simulink model "ACDCMG_sim8"  (R2019b)
settings: Solver=ode8  StartTime=0.0  StopTime=0.5  FixedStep=40e-6  MaxStep=1e-2  RelTol=1e-3
PreLoadFcn:
  | Set_parameters_R2018
InitFcn:
  | Set_parameters_R2018
values from neighbouring files (symbols this model uses):
  dis11 = 3    [Set_parameters_R2018.m]
  dis12 = 3    [Set_parameters_R2018.m]
  dis2 = 0.2    [Set_parameters_R2018.m]
  dis3 = 0.15    [Set_parameters_R2018.m]
  dis4 = 0.2    [Set_parameters_R2018.m]
  dis5 = 0.25    [Set_parameters_R2018.m]
  dis6 = 0.1    [Set_parameters_R2018.m]
  Fnom = 60    [Set_parameters_R2018.m]
  max_min = 1    [Set_parameters_R2018.m]
  P_Load_3 = S_Load_3* PF_Load_3    (= 7650)    [Set_parameters_R2018.m]
  Pnom_T1 = 1.5e6    (= 1500000)    [Set_parameters_R2018.m]
  Pnom_T2 = 1.5e6    (= 1500000)    [Set_parameters_R2018.m]
  Pnom_T3 = 4e6    (= 4000000)    [Set_parameters_R2018.m]
  Ql_Load_3 = S_Load_3 * sin(acos(PF_Load_3))    [Set_parameters_R2018.m]
  R_Load_9 = (Vnom_prim * 1.35)^2 / P_Load_9    (= 1084.6153125)    [Set_parameters_R2018.m]
  R_Load_DC = Vnom_DC^2/ P_Load_DC    (= 45)    [Set_parameters_R2018.m]
  Rl = 0.17    [Set_parameters_R2018.m]
  Rls = 0.013    [Set_parameters_R2018.m]
  Ts = 40e-6    (= 4e-05)    [Set_parameters_R2018.m]
  Ts_Control = 6*Ts_Power    (= 0.00024)    [Set_parameters_R2018.m]
  Ts_Power = Ts    (= 4e-05)    [Set_parameters_R2018.m]
  Ts_PV = 0.05    [Set_parameters_R2018.m]
  V1_LL_T3 = 69e3    (= 69000)    [Set_parameters_R2018.m]
  Vmin_mppt = 100    [Set_parameters_R2018.m]
  Vnom_DC = 300    [Set_parameters_R2018.m]
  Vnom_Diesel = 2.4e3    (= 2400)    [Set_parameters_R2018.m]
  Vnom_prim = 13.8e3    (= 13800)    [Set_parameters_R2018.m]
  Vnom_sec = 220    [Set_parameters_R2018.m]
  Vnom_ter_AC_DC = 150    [Set_parameters_R2018.m]
  Xl = 0.3    [Set_parameters_R2018.m]
  Xls = 0.93e-3    (= 0.00093)    [Set_parameters_R2018.m]
undefined symbols (not defined in the file or in its folder): D1, Delta, DiscIntNeverNeededParam, fn, Ion, Lithium, VnInv
libraries: powerlib x136, powerlib_meascontrol x67, rtlab x23, artemis x7, simulink x7, powerlib_extras x5, electricdrivelib x1, eeSinusoidalMeasurementV2 x1, op_dpl_lib x1, re_lib x1
(part 4 of 5)

== system ACDCMG_sim8/SM_Grid_Simulation/Boost -buck Bi-directional converter 1/Primary Control ==
  V_ref : Inport
  Constant : Constant
  Display3 : Display  Commented=on
  From1 : From  Commented=on  GotoTag=Vdc_bus  TagVisibility=global
  From4 : From  Commented=on  GotoTag=boost1
  From5 : From  Commented=on  GotoTag=buck1
  PID Orig Boost : Subsystem
  Relational Operator2 : RelationalOperator  Commented=on  Operator=>  OutDataTypeStr=boolean  RndMeth=Nearest
  Saturation : Saturate  UpperLimit=0.9  LowerLimit=0.1
  Sum : Sum  Inputs=|+-
  Sum1 : Sum  Inputs=|-+
  Switch : Switch  Commented=on  Criteria=u2 > Threshold  Threshold=300
  Switch1 : Switch  Commented=on  Criteria=u2 > Threshold  Threshold=300
  Vref1 : Constant  Commented=on  Value=0
  Vref2 : Constant  Commented=on  Value=0
  Duty_Ctrl : Outport  VectorParamsAs1DForOutWhenUnconnected=off
  Comp_Duty_Ctrl : Outport  Port=2  VectorParamsAs1DForOutWhenUnconnected=off
  wires:
  Relational Operator2/1 -> Switch1/2, Switch/2
  V_ref/1 -> Sum/1, Relational Operator2/2
  From1/1 -> Relational Operator2/1
  Vref2/1 -> Switch1/1
  [V_DC_bus_BESS] -> Sum/2
  From5/1 -> Switch/1
  From4/1 -> Switch1/3
  Switch/1 -> Display3/1
  Vref1/1 -> Switch/3
  Sum/1 -> PID Orig Boost/1(error)  "error"
  PID Orig Boost/1(Out1) -> Saturation/1
  Constant/1 -> Sum1/2
  Saturation/1 -> Sum1/1, Duty_Ctrl/1
  Sum1/1 -> Comp_Duty_Ctrl/1

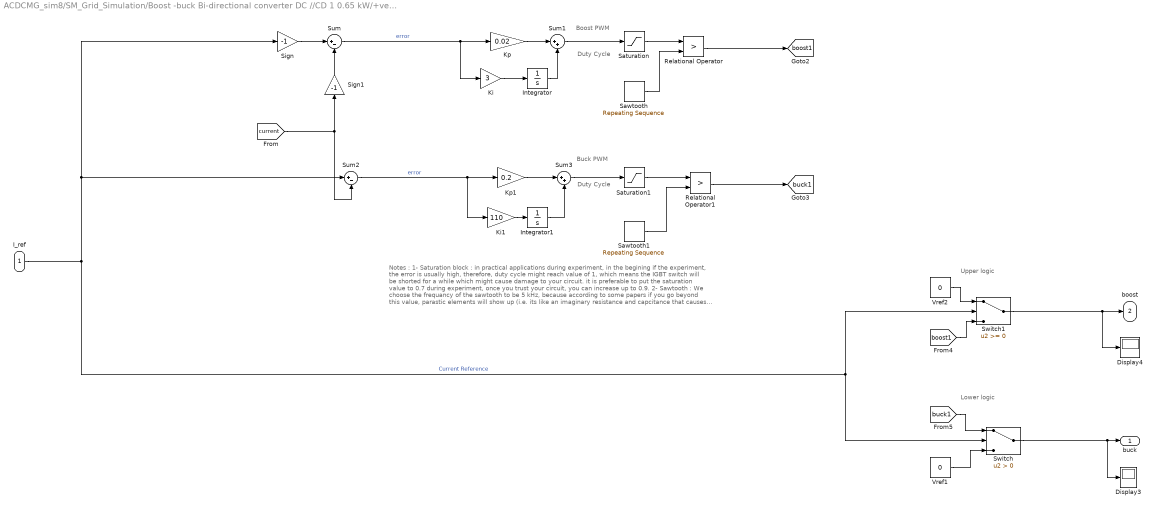
== system ACDCMG_sim8/SM_Grid_Simulation/Boost -buck Bi-directional converter DC //CD 1 0.65 kW/+ve reference For Buck --> -ve reference For Boost <-- ==
  note: Notes :
      | 1- Saturation block : in practical applications during experiment, in the begining if the experiment, the error is usually high, therefore, duty cycle might reach value of 1, which means the IGBT switch will be shorted for a while which might cause damage to your circuit. it is preferable to put the saturation value to 0.7 during experiment, once you trust your circuit, you can increase up to 0.9.
      | 2- Sawtooth : We choose the frequancy of the sawtooth to be 5 kHz, because according to some papers if you go beyond this value, parastic elements will show up (i.e. its like an imaginary resistance and capcitance that causes switching losses and heat). But the more you increase the frequency, the smoother the signal you will get.
      | 3- Step size of your mode l: Make sure that the step size (sample time) in the "model configuration parameters" is smaller than 1/f of the sawtooth. For example, lets say that the sawtooth f = 2 Hz or cycle/sec, meaning the triangle (cycle) repeats every 1/2 sec. Step size or sample time means how many point matlab plot every cycle, lets say it is 1/4 (i.e. plot a point every 0.25 sec), that means that the triangle will be plotted with only two points. That reduce the accuracy, Moreover if the step size is greater than 1/f of the sawtooth, the sawtooth output will be zero.
  note: Buck PWM
  note: Duty Cycle
  note: Upper logic
  note: Lower logic
  note: Boost PWM
  note: Duty Cycle
  I_ref : Inport
  Display3 : Display
  Display4 : Display
  Integrator : Integrator  LimitOutput=on  UpperSaturationLimit=0.9  LowerSaturationLimit=0
  Integrator1 : Integrator  LimitOutput=on  UpperSaturationLimit=0.9  LowerSaturationLimit=0
  Ki : Gain  Gain=3
  Ki1 : Gain  Gain=110
  Kp : Gain  Gain=0.02
  Kp1 : Gain  Gain=0.2
  Relational Operator : RelationalOperator  Operator=>  OutDataTypeStr=boolean  RndMeth=Nearest
  Relational Operator1 : RelationalOperator  Operator=>  OutDataTypeStr=boolean  RndMeth=Nearest
  Saturation : Saturate  UpperLimit=0.9  LowerLimit=0
  Saturation1 : Saturate  UpperLimit=0.8  LowerLimit=0
  Sawtooth : simulink/Sources/Repeating Sequence  rep_seq_t=[0 1/5000]  rep_seq_y=[0 1]
  Sawtooth1 : simulink/Sources/Repeating Sequence  rep_seq_t=[0 1/5000]  rep_seq_y=[0 1]
  Sign : Gain  Gain=-1
  Sign1 : Gain  Gain=-1
  Sum : Sum  Inputs=|+-
  Sum1 : Sum  Inputs=|++
  Sum2 : Sum  Inputs=|+-
  Sum3 : Sum  Inputs=|++
  Switch : Switch  Criteria=u2 > Threshold
  Switch1 : Switch
  Vref1 : Constant  Value=0
  Vref2 : Constant  Value=0
  buck : Outport  VectorParamsAs1DForOutWhenUnconnected=off
  boost : Outport  Port=2  VectorParamsAs1DForOutWhenUnconnected=off
  tag scope: boost1=global, buck1=global
  wires:
  Integrator/1 -> Sum1/2
  Kp/1 -> Sum1/1
  Sum/1 -> Kp/1, Ki/1  "error"
  Relational Operator/1 -> [boost1]
  Sign/1 -> Sum/1
  Sum1/1 -> Saturation/1
  Ki/1 -> Integrator/1
  Sum3/1 -> Saturation1/1
  Integrator1/1 -> Sum3/2
  Sawtooth/1 -> Relational Operator/2
  Sawtooth1/1 -> Relational Operator1/2
  [current] -> Sum2/2, Sign1/1
  Kp1/1 -> Sum3/1
  Relational Operator1/1 -> [buck1]
  Sum2/1 -> Ki1/1, Kp1/1  "error"
  Saturation/1 -> Relational Operator/1
  Saturation1/1 -> Relational Operator1/1
  Ki1/1 -> Integrator1/1
  Vref1/1 -> Switch/3
  Vref2/1 -> Switch1/1
  [boost1] -> Switch1/3
  [buck1] -> Switch/1
  I_ref/1 -> Sum2/1, Sign/1, Switch1/2, Switch/2  "Current Reference"
  Sign1/1 -> Sum/2
  Switch1/1 -> Display4/1, boost/1
  Switch/1 -> Display3/1, buck/1

== system ACDCMG_sim8/SM_Grid_Simulation/Boost -buck Bi-directional converter DC //CD 1 0.65 kW/ref ==
  note: 1 -charge
      | 0-discharge
  Constant2 : Constant  Value=max_min
  Constant3 : Constant  Value=max_min
  Current reference (battery charge) OP_Max : Constant  Value=5
  Current reference (battery discharge) OP_Max1 : Constant  Value=-5
  Min Demand OP_min : Constant  Value=3
  Min Demand OP_min1 : Constant  Value=-3
  Switch : Switch  Criteria=u2 > Threshold
  Switch1 : Switch  Criteria=u2 > Threshold
  Switch3 : Switch  Criteria=u2 > Threshold
  Vref1 : Constant
  ref : Outport  VectorParamsAs1DForOutWhenUnconnected=off
  wires:
  Constant3/1 -> Switch3/2
  Switch3/1 -> Switch/3
  Switch1/1 -> Switch/1
  Vref1/1 -> Switch/2
  Min Demand OP_min/1 -> Switch1/3
  Current reference (battery charge) OP_Max/1 -> Switch1/1
  Min Demand OP_min1/1 -> Switch3/3
  Constant2/1 -> Switch1/2
  Current reference (battery discharge) OP_Max1/1 -> Switch3/1
  Switch/1 -> ref/1

== system ACDCMG_sim8/SM_Grid_Simulation/Boost converter 2 5 kHz - 300V /MPPT Controller using  Incremental Conductance and Integral Regulator  technique  ==
  note: +
  note: control mppt
  V_PV : Inport
  I_PV : Inport  Port=2
  Add : Sum
  Deblock MPPT : Step  Time=Ts_PV  Before=-1  SampleTime=0
  Duty Cycle : Constant  Commented=on  Value=Dinit
  Goto7 : Goto  Commented=on  GotoTag=D  TagVisibility=global
  MPPT : Subsystem
  PWM Generator (DC-DC) : powerlib_meascontrol/Pulse & Signal Generators/PWM Generator (DC-DC)  Commented=on  Fsw=fc  Ts=Ts_Power
  Saturation : Saturate  UpperLimit=0.9  LowerLimit=0.1
  Pulses : Outport  VectorParamsAs1DForOutWhenUnconnected=off
  wires:
  V_PV/1 -> MPPT/1(V_PV)
  I_PV/1 -> MPPT/2(I_PV)
  Deblock MPPT/1 -> MPPT/3(on/off)
  Add/1 -> Saturation/1  "D"
  MPPT/1(D) -> Add/2  "Vdc_ref"
  Saturation/1 -> Pulses/1

== system ACDCMG_sim8/SM_Grid_Simulation/Bus_1/Power Factor Block1 ==
  Vabc : Inport
  Iabc : Inport  Port=2
  Complex to Magnitude-Angle : ComplexToMagnitudeAngle  Commented=on
  Conv pu2 : Gain  Gain=1/Vnom_Diesel  SaturateOnIntegerOverflow=on  OutDataTypeStr=Inherit: Same as input  ParamDataTypeStr=Inherit: Same as input
  Current3 : Goto  Commented=on  GotoTag=P_abc_Bus8  TagVisibility=global
  Current4 : Goto  Commented=on  GotoTag=Q_abc_Bus8  TagVisibility=global
  Gain : Gain  Commented=on  Gain=-1/1000
  Gain1 : Gain  Commented=on  Gain=-1/1000
  Memory : Memory
  Power : powerlib_meascontrol/Measurements/Power  Commented=on  Freq=Freq  Vinit=Vinit  Iinit=Iinit  Ts=Ts
  RMS : powerlib_meascontrol/Measurements/RMS  TrueRMS=on  Freq=60  RMSInit=120  Ts=0
  Real-Imag to Complex : RealImagToComplex  Commented=on
  Terminator : Terminator  Commented=on
  cos(theta) : Trigonometry  Commented=on  Operator=cos
  "Vabc y Vabc " : Outport  VectorParamsAs1DForOutWhenUnconnected=off
  "Iabc y Iabc " : Outport  Port=2  VectorParamsAs1DForOutWhenUnconnected=off
  tag scope: Vabc_LL_pu_Bus1=global
  wires:
  Complex to Magnitude-Angle/2 -> cos(theta)/1
  Real-Imag to Complex/1 -> Complex to Magnitude-Angle/1
  cos(theta)/1 -> ?
  Complex to Magnitude-Angle/1 -> Terminator/1
  Iabc/1 -> "Iabc y Iabc "/1, Power/2
  Vabc/1 -> Memory/1, Power/1
  Power/2 -> Real-Imag to Complex/2, Gain/1
  Power/1 -> Gain1/1, Real-Imag to Complex/1
  Gain/1 -> Current4/1
  Gain1/1 -> Current3/1
  RMS/1 -> Conv pu2/1
  Conv pu2/1 -> [Vabc_LL_pu_Bus1]
  Memory/1 -> RMS/1, "Vabc y Vabc "/1

== system ACDCMG_sim8/SM_Grid_Simulation/Bus_2/Power Factor Block1 ==
  Vabc : Inport
  Iabc : Inport  Port=2
  Complex to Magnitude-Angle : ComplexToMagnitudeAngle  Commented=on
  Conv pu1 : Gain  Gain=1/Vnom_sec  SaturateOnIntegerOverflow=on  OutDataTypeStr=Inherit: Same as input  ParamDataTypeStr=Inherit: Same as input
  Current1 : Goto  Commented=on  GotoTag=P_abc_Bus1  TagVisibility=global
  Current2 : Goto  Commented=on  GotoTag=Q_abc_Bus1  TagVisibility=global
  Gain1 : Gain  Commented=on  Gain=-1/1000
  Memory : Memory
  Mux : Mux  Inputs=1
  Power : powerlib_meascontrol/Measurements/Power  Commented=on  Freq=Freq  Vinit=Vinit  Iinit=Iinit  Ts=Ts
  RMS : powerlib_meascontrol/Measurements/RMS  TrueRMS=on  Freq=60  RMSInit=120  Ts=0
  Real-Imag to Complex : RealImagToComplex  Commented=on
  Terminator : Terminator  Commented=on
  cos(theta) : Trigonometry  Commented=on  Operator=cos
  to Kw : Gain  Commented=on  Gain=-1/1000
  "Vabc y Vabc " : Outport  VectorParamsAs1DForOutWhenUnconnected=off
  "Iabc y Iabc " : Outport  Port=2  VectorParamsAs1DForOutWhenUnconnected=off
  tag scope: Vabc_LL_pu_Bus2=global
  wires:
  Power/1 -> Gain1/1, Real-Imag to Complex/1
  Power/2 -> Real-Imag to Complex/2, to Kw/1
  Complex to Magnitude-Angle/2 -> cos(theta)/1
  Real-Imag to Complex/1 -> Complex to Magnitude-Angle/1
  Complex to Magnitude-Angle/1 -> Terminator/1
  Iabc/1 -> "Iabc y Iabc "/1, Power/2
  Mux/1 -> "Vabc y Vabc "/1
  Vabc/1 -> Power/1, Memory/1
  to Kw/1 -> Current2/1
  Gain1/1 -> Current1/1
  RMS/1 -> Conv pu1/1
  Conv pu1/1 -> [Vabc_LL_pu_Bus2]
  Memory/1 -> Mux/1, RMS/1

== system ACDCMG_sim8/SM_Grid_Simulation/Bus_3/Power Factor Block1 ==
  Vabc : Inport
  Iabc : Inport  Port=2
  Complex to Magnitude-Angle : ComplexToMagnitudeAngle  Commented=on
  Conv pu1 : Gain  Gain=1/Vnom_sec  SaturateOnIntegerOverflow=on  OutDataTypeStr=Inherit: Same as input  ParamDataTypeStr=Inherit: Same as input
  Current3 : Goto  Commented=on  GotoTag=P_abc_Bus4  TagVisibility=global
  Current4 : Goto  Commented=on  GotoTag=Q_abc_Bus4  TagVisibility=global
  Memory : Memory
  Mux : Mux  Inputs=1
  Power : powerlib_meascontrol/Measurements/Power  Commented=on  Freq=Freq  Vinit=Vinit  Iinit=Iinit  Ts=Ts
  RMS : powerlib_meascontrol/Measurements/RMS  TrueRMS=on  Freq=60  RMSInit=120  Ts=0
  Real-Imag to Complex : RealImagToComplex  Commented=on
  Terminator : Terminator  Commented=on
  cos(theta) : Trigonometry  Commented=on  Operator=cos
  to Kw : Gain  Commented=on  Gain=1/1000
  to Kw1 : Gain  Commented=on  Gain=1/1000
  Vabc y Vabc : Outport  VectorParamsAs1DForOutWhenUnconnected=off
  "Iabc y Iabc " : Outport  Port=2  VectorParamsAs1DForOutWhenUnconnected=off
  tag scope: Vabc_LL_pu_Bus3=global
  wires:
  Complex to Magnitude-Angle/2 -> cos(theta)/1
  Real-Imag to Complex/1 -> Complex to Magnitude-Angle/1
  cos(theta)/1 -> ?
  Complex to Magnitude-Angle/1 -> Terminator/1
  Iabc/1 -> "Iabc y Iabc "/1, Power/2
  Mux/1 -> Vabc y Vabc/1
  Vabc/1 -> Power/1, Memory/1
  Power/2 -> Real-Imag to Complex/2, to Kw/1
  Power/1 -> to Kw1/1, Real-Imag to Complex/1
  to Kw/1 -> Current4/1
  to Kw1/1 -> Current3/1
  RMS/1 -> Conv pu1/1
  Conv pu1/1 -> [Vabc_LL_pu_Bus3]
  Memory/1 -> Mux/1, RMS/1

== system ACDCMG_sim8/SM_Grid_Simulation/Bus_4/Power Factor Block1 ==
  Vabc : Inport
  Iabc : Inport  Port=2
  Complex to Magnitude-Angle : ComplexToMagnitudeAngle  Commented=on
  Conv pu1 : Gain  Gain=1/Vnom_sec  SaturateOnIntegerOverflow=on  OutDataTypeStr=Inherit: Same as input  ParamDataTypeStr=Inherit: Same as input
  Current3 : Goto  Commented=on  GotoTag=P_abc_Bus4  TagVisibility=global
  Current4 : Goto  Commented=on  GotoTag=Q_abc_Bus4  TagVisibility=global
  Memory : Memory
  Mux : Mux  Inputs=1
  Power : powerlib_meascontrol/Measurements/Power  Commented=on  Freq=Freq  Vinit=Vinit  Iinit=Iinit  Ts=Ts
  RMS : powerlib_meascontrol/Measurements/RMS  TrueRMS=on  Freq=60  RMSInit=120  Ts=0
  Real-Imag to Complex : RealImagToComplex  Commented=on
  Terminator : Terminator  Commented=on
  cos(theta) : Trigonometry  Commented=on  Operator=cos
  to Kw : Gain  Commented=on  Gain=1/1000
  to Kw1 : Gain  Commented=on  Gain=1/1000
  Vabc y Vabc : Outport  VectorParamsAs1DForOutWhenUnconnected=off
  "Iabc y Iabc " : Outport  Port=2  VectorParamsAs1DForOutWhenUnconnected=off
  tag scope: Vabc_LL_pu_Bus4=global
  wires:
  Complex to Magnitude-Angle/2 -> cos(theta)/1
  Real-Imag to Complex/1 -> Complex to Magnitude-Angle/1
  cos(theta)/1 -> ?
  Complex to Magnitude-Angle/1 -> Terminator/1
  Iabc/1 -> "Iabc y Iabc "/1, Power/2
  Mux/1 -> Vabc y Vabc/1
  Vabc/1 -> Power/1, Memory/1
  Power/2 -> Real-Imag to Complex/2, to Kw/1
  Power/1 -> to Kw1/1, Real-Imag to Complex/1
  to Kw/1 -> Current4/1
  to Kw1/1 -> Current3/1
  RMS/1 -> Conv pu1/1
  Conv pu1/1 -> [Vabc_LL_pu_Bus4]
  Memory/1 -> Mux/1, RMS/1

== system ACDCMG_sim8/SM_Grid_Simulation/Bus_5/Power Factor Block1 ==
  Vabc : Inport
  Iabc : Inport  Port=2
  Complex to Magnitude-Angle : ComplexToMagnitudeAngle  Commented=on
  Conv pu1 : Gain  Gain=1/Vnom_sec  SaturateOnIntegerOverflow=on  OutDataTypeStr=Inherit: Same as input  ParamDataTypeStr=Inherit: Same as input
  Current3 : Goto  Commented=on  GotoTag=P_abc_Bus5  TagVisibility=global
  Current4 : Goto  Commented=on  GotoTag=Q_abc_Bus5  TagVisibility=global
  Memory : Memory
  Mux : Mux  Inputs=2
  Power : powerlib_meascontrol/Measurements/Power  Commented=on  Freq=Freq  Vinit=Vinit  Iinit=Iinit  Ts=Ts
  RMS : powerlib_meascontrol/Measurements/RMS  TrueRMS=on  Freq=60  RMSInit=120  Ts=0
  Real-Imag to Complex : RealImagToComplex  Commented=on
  Terminator : Terminator  Commented=on
  cos(theta) : Trigonometry  Commented=on  Operator=cos
  to Kw : Gain  Commented=on  Gain=1/1000
  to Kw1 : Gain  Commented=on  Gain=1/1000
  Vabc y Vabc : Outport  VectorParamsAs1DForOutWhenUnconnected=off
  "Iabc y Iabc " : Outport  Port=2  VectorParamsAs1DForOutWhenUnconnected=off
  tag scope: Vabc_LL_pu_Bus5=global
  wires:
  Complex to Magnitude-Angle/2 -> cos(theta)/1
  Real-Imag to Complex/1 -> Complex to Magnitude-Angle/1
  cos(theta)/1 -> ?
  Complex to Magnitude-Angle/1 -> Terminator/1
  Iabc/1 -> "Iabc y Iabc "/1, Power/2
  Mux/1 -> Vabc y Vabc/1
  Vabc/1 -> Power/1, Memory/1
  Power/2 -> Real-Imag to Complex/2, to Kw/1
  Power/1 -> to Kw1/1, Real-Imag to Complex/1
  to Kw/1 -> Current4/1
  to Kw1/1 -> Current3/1
  RMS/1 -> Conv pu1/1
  Conv pu1/1 -> [Vabc_LL_pu_Bus5]
  Memory/1 -> RMS/1, Mux/2

== system ACDCMG_sim8/SM_Grid_Simulation/Bus_6/Power Factor Block1 ==
  Vabc : Inport
  Iabc : Inport  Port=2
  Complex to Magnitude-Angle : ComplexToMagnitudeAngle  Commented=on
  Conv pu1 : Gain  Gain=1/Vnom_sec  SaturateOnIntegerOverflow=on  OutDataTypeStr=Inherit: Same as input  ParamDataTypeStr=Inherit: Same as input
  Current3 : Goto  Commented=on  GotoTag=P_abc_Bus2  TagVisibility=global
  Current4 : Goto  Commented=on  GotoTag=Q_abc_Bus2  TagVisibility=global
  Memory : Memory
  Mux : Mux  Inputs=1
  Power : powerlib_meascontrol/Measurements/Power  Commented=on  Freq=Freq  Vinit=Vinit  Iinit=Iinit  Ts=Ts
  RMS : powerlib_meascontrol/Measurements/RMS  TrueRMS=on  Freq=60  RMSInit=120  Ts=0
  Real-Imag to Complex : RealImagToComplex  Commented=on
  Terminator : Terminator  Commented=on
  cos(theta) : Trigonometry  Commented=on  Operator=cos
  to Kw : Gain  Commented=on  Gain=-1/1000
  to Kw1 : Gain  Commented=on  Gain=-1/1000
  "Vabc y Vabc " : Outport  VectorParamsAs1DForOutWhenUnconnected=off
  Iabc y Iabc : Outport  Port=2  VectorParamsAs1DForOutWhenUnconnected=off
  tag scope: Vabc_LL_pu_Bus6=global
  wires:
  Complex to Magnitude-Angle/2 -> cos(theta)/1
  Real-Imag to Complex/1 -> Complex to Magnitude-Angle/1
  cos(theta)/1 -> ?
  Complex to Magnitude-Angle/1 -> Terminator/1
  Iabc/1 -> Iabc y Iabc/1, Power/2
  Mux/1 -> "Vabc y Vabc "/1
  Vabc/1 -> Power/1, Memory/1
  Power/1 -> to Kw1/1, Real-Imag to Complex/1
  Power/2 -> to Kw/1, Real-Imag to Complex/2
  to Kw/1 -> Current4/1
  to Kw1/1 -> Current3/1
  RMS/1 -> Conv pu1/1
  Conv pu1/1 -> [Vabc_LL_pu_Bus6]
  Memory/1 -> Mux/1, RMS/1

== system ACDCMG_sim8/SM_Grid_Simulation/Bus_7/Power Factor Block1 ==
  Vabc : Inport
  Iabc : Inport  Port=2
  Complex to Magnitude-Angle : ComplexToMagnitudeAngle  Commented=on
  Conv pu1 : Gain  Gain=1/Vnom_sec  SaturateOnIntegerOverflow=on  OutDataTypeStr=Inherit: Same as input  ParamDataTypeStr=Inherit: Same as input
  Memory : Memory
  Power : powerlib_meascontrol/Measurements/Power  Commented=on  Freq=Freq  Vinit=Vinit  Iinit=Iinit  Ts=Ts
  RMS : powerlib_meascontrol/Measurements/RMS  TrueRMS=on  Freq=60  RMSInit=120  Ts=0
  Real-Imag to Complex : RealImagToComplex  Commented=on
  Terminator : Terminator  Commented=on
  cos(theta) : Trigonometry  Commented=on  Operator=cos
  Vabc y Vabc : Outport  VectorParamsAs1DForOutWhenUnconnected=off
  "Iabc y Iabc " : Outport  Port=2  VectorParamsAs1DForOutWhenUnconnected=off
  tag scope: Vabc_LL_pu_Bus7=global
  wires:
  Power/1 -> Real-Imag to Complex/1
  Power/2 -> Real-Imag to Complex/2
  Complex to Magnitude-Angle/2 -> cos(theta)/1
  Real-Imag to Complex/1 -> Complex to Magnitude-Angle/1
  cos(theta)/1 -> ?
  Complex to Magnitude-Angle/1 -> Terminator/1
  Iabc/1 -> "Iabc y Iabc "/1, Power/2
  Vabc/1 -> Memory/1, Power/1
  RMS/1 -> Conv pu1/1
  Conv pu1/1 -> [Vabc_LL_pu_Bus7]
  Memory/1 -> RMS/1, Vabc y Vabc/1

== system ACDCMG_sim8/SM_Grid_Simulation/Bus_8/Power Factor Block1 ==
  Vabc : Inport
  Iabc : Inport  Port=2
  Complex to Magnitude-Angle : ComplexToMagnitudeAngle  Commented=on
  Conv pu1 : Gain  Gain=1/Vnom_ter_AC_DC  SaturateOnIntegerOverflow=on  OutDataTypeStr=Inherit: Same as input  ParamDataTypeStr=Inherit: Same as input
  Memory1 : Memory
  Power : powerlib_meascontrol/Measurements/Power  Commented=on  Freq=Freq  Vinit=Vinit  Iinit=Iinit  Ts=Ts
  RMS : powerlib_meascontrol/Measurements/RMS  TrueRMS=on  Freq=60  RMSInit=120  Ts=0
  Real-Imag to Complex : RealImagToComplex  Commented=on
  Terminator : Terminator  Commented=on
  cos(theta) : Trigonometry  Commented=on  Operator=cos
  "Vabc y Vabc " : Outport  VectorParamsAs1DForOutWhenUnconnected=off
  "Iabc y Iabc " : Outport  Port=2  VectorParamsAs1DForOutWhenUnconnected=off
  tag scope: Vabc_LL_pu_Bus8=global
  wires:
  Power/1 -> Real-Imag to Complex/1
  Power/2 -> Real-Imag to Complex/2
  Complex to Magnitude-Angle/2 -> cos(theta)/1
  Real-Imag to Complex/1 -> Complex to Magnitude-Angle/1
  cos(theta)/1 -> ?
  Complex to Magnitude-Angle/1 -> Terminator/1
  Iabc/1 -> "Iabc y Iabc "/1, Power/2
  Vabc/1 -> Memory1/1, Power/1
  RMS/1 -> Conv pu1/1
  Conv pu1/1 -> [Vabc_LL_pu_Bus8]
  Memory1/1 -> "Vabc y Vabc "/1, RMS/1

== system ACDCMG_sim8/SM_Grid_Simulation/Bus_AC//DC3/Battery system ==
  note: DC Bus (port)
  note: Battery (port)
  "0 = Enable (Do it after transient, so that it does not calculate ripples during transient) 1 = Reset after every change in current reference" : Constant  Commented=on  Value=0
  Current Inst : Scope
  Current going to/ from the battery : Scope
  Mean : powerlib_meascontrol/Measurements/Mean  Freq=10  Vinit=0  Ts=Ts_Power
  Power : Product
  Power Bess1 : Scope
  Power Bus : Scope
  Power1 : Product
  Ripple Calculations : Subsystem  Commented=on
  Ripple in Boost : Display  Commented=on
  Ripple in Buck : Display  Commented=on
  Vbat : Scope
  Vdc : Scope
  to Kw : Gain  Gain=1/1000
  to Kw1 : Gain  Gain=1/1000
  tag scope: DC_Bus_Power=global, Ibat=global, Power_Bess1=global, Vbat=global
  wires:
  to Kw/1 -> [DC_Bus_Power], Power Bus/1
  Mean/1 -> Power/2
  Power/1 -> to Kw/1
  Ripple Calculations/1(Ripple in Buck) -> Ripple in Buck/1
  "0 = Enable (Do it after transient, so that it does not calculate ripples during transient) 1 = Reset after every change in current reference"/1 -> Ripple Calculations/2(Reset)
  Ripple Calculations/2(Ripple in Boost) -> Ripple in Boost/1
  [I_DC_bus_BESS] -> Current Inst/1, Mean/1, Ripple Calculations/1(Signal)
  [Idc_battery] -> Power1/2, [Ibat], Current going to/ from the battery/1
  [V_DC_bus_BESS] -> Vdc/1, Power/1
  [Vdc_battery] -> Power1/1, [Vbat], Vbat/1
  to Kw1/1 -> [Power_Bess1], Power Bess1/1
  Power1/1 -> to Kw1/1

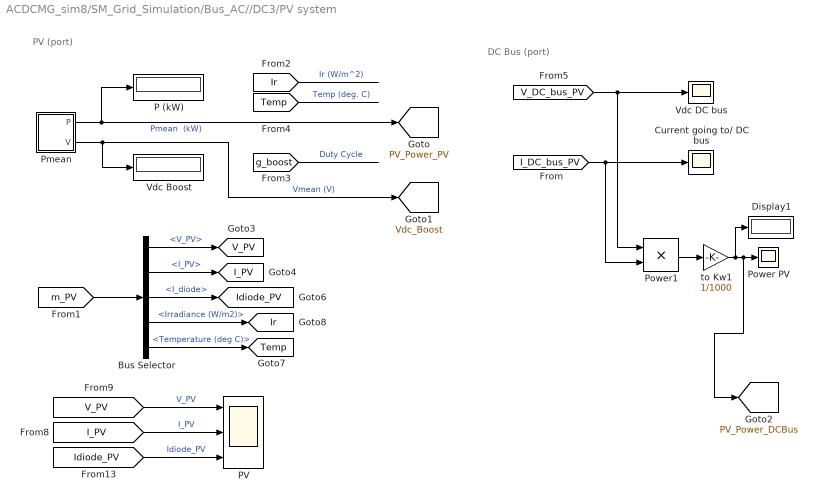
== system ACDCMG_sim8/SM_Grid_Simulation/Bus_AC//DC3/PV system ==
  note: PV (port)
  note: DC Bus (port)
  Bus Selector : BusSelector  OutputSignals=V_PV,I_PV,I_diode,Irradiance (W/m2),Temperature (deg C)
  Current going to/ DC bus : Scope
  Display1 : Display
  "P (kW) " : Display
      settings: Format=bank  Decimation=2000
  PV : Scope  NumInputPorts=3
  Pmean : Subsystem
  Power PV : Scope
  Power1 : Product
  Vdc Boost : Display
      settings: Format=bank  Decimation=2000
  Vdc DC bus : Scope
  to Kw1 : Gain  Gain=1/1000
  tag scope: I_PV=global, Idiode_PV=global, Ir=global, PV_Power_DCBus=global, PV_Power_PV=global, Temp=global, V_PV=global, Vdc_Boost=global
  wires:
  [V_PV] -> PV/1  "V_PV"
  [I_PV] -> PV/2  "I_PV"
  [Idiode_PV] -> PV/3  "Idiode_PV"
  [m_PV] -> Bus Selector/1
  Bus Selector/1 -> [V_PV]  "<V_PV>"
  Bus Selector/2 -> [I_PV]  "<I_PV>"
  Bus Selector/4 -> [Ir]  "<Irradiance (W/m2)>"
  Bus Selector/3 -> [Idiode_PV]  "<I_diode>"
  Bus Selector/5 -> [Temp]  "<Temperature (deg C)>"
  [Temp] -> ?  "Temp (deg. C)"
  [g_boost] -> ?  "Duty Cycle"
  Pmean/2(V) -> [Vdc_Boost], Vdc Boost/1  "Vmean (V)"
  [Ir] -> ?  "Ir (W/m^2)"
  Pmean/1(P) -> [PV_Power_PV], "P (kW) "/1  "Pmean  (kW)"
  [V_DC_bus_PV] -> Vdc DC bus/1, Power1/1
  [I_DC_bus_PV] -> Power1/2, Current going to/ DC bus/1
  to Kw1/1 -> Display1/1, [PV_Power_DCBus], Power PV/1
  Power1/1 -> to Kw1/1

== system ACDCMG_sim8/SM_Grid_Simulation/DATA  ADQUISITION/Power_Losses_abc ==
  From10 : From  Commented=on  GotoTag=Power_Losse_abc_L10  TagVisibility=global
  From11 : From  Commented=on  GotoTag=Power_Losse_abc_L10
  From12 : From  Commented=on  GotoTag=Power_Losse_abc_L12
  From13 : From  Commented=on  GotoTag=Power_Losse_abc_L14
  From6 : From  Commented=on  GotoTag=Power_Losse_abc_L3  TagVisibility=global
  From8 : From  Commented=on  GotoTag=Power_Losse_abc_L8  TagVisibility=global
  From9 : From  Commented=on  GotoTag=Power_Losse_abc_L9  TagVisibility=global
  Mux : Mux  Inputs=7
  f2 : ToWorkspace  VariableName=Power_Losse_abc  SaveFormat=Timeseries  SampleTime=-1
  wires:
  [Power_Losse_abc_L1] -> Mux/1
  Mux/1 -> f2/1
  [Power_Losse_abc_L2] -> Mux/2
  [Power_Losse_abc_L5] -> Mux/5
  [Power_Losse_abc_L6] -> Mux/6
  [Power_Losse_abc_L7] -> Mux/7
  [Power_Losse_abc_L3] -> Mux/3
  [Power_Losse_abc_L4] -> Mux/4

== system ACDCMG_sim8/SM_Grid_Simulation/DATA  ADQUISITION/VoltageLL_pu_abc ==
  From25 : From  Commented=on  GotoTag=Vabc_LL_pu_Bus9  TagVisibility=global
  From28 : From  Commented=on  GotoTag=Vabc_LL_pu_Bus10
  From31 : From  Commented=on  GotoTag=Vabc_LL_pu_Bus10
  From34 : From  Commented=on  GotoTag=Vabc_LL_pu_Bus12
  From40 : From  Commented=on  GotoTag=Vabc_LL_pu_Bus14
  Mux : Mux  Inputs=9
  f2 : ToWorkspace  VariableName=VoltageLL_pu_abc  SaveFormat=Timeseries  SampleTime=-1
  wires:
  [Vabc_LL_pu_Bus4] -> Mux/4
  [Vabc_LL_pu_Bus5] -> Mux/5
  Mux/1 -> f2/1
  [Vabc_LL_pu_Bus8] -> Mux/8
  [Vabc_LL_pu_Bus1] -> Mux/1
  [Vabc_LL_pu_Bus2] -> Mux/2
  [Vabc_LL_pu_Bus6] -> Mux/6
  [Vabc_LL_pu_Bus7] -> Mux/7
  [V_pu_BusDC] -> Mux/9
  [Vabc_LL_pu_Bus3] -> Mux/3

== system ACDCMG_sim8/SM_Grid_Simulation/Grid Bi-directional Converter 1.1 300 (DC) // 150 V (AC) P_nom 3kW2/Control of Inverter ==
  note: VL-L rms_1
  note: Primary control
  note: Control of Inverter
  Means : Inport
  Bus Selector : BusSelector  OutputSignals=signal1,signal2,signal3,signal4
  Discrete PWM Generator1 : Subsystem  AncestorBlock=|  DialogController=POWERSYS.PowerSysDialog  mask(Discrete PWM Generator){GeneratorMode=3-arm  bridge (6 pulses), Fc=4000, Ts=Ts_Power, Internal=off, mIndex=0.99, Freq=60, Phase=0}
      | powerlib_extras/Discrete 
      | Control Blocks/Discrete
      | PWM Generator
      mask prompts: GeneratorMode "Generator Mode"; Fc "Carrier frequency (Hz):"; Ts "Sample time:"; Internal "Internal generation of modulating signal(s)"; mIndex "Modulation index  (0<m<1) :"; Freq "Frequency of output voltage (Hz)"; Phase "Phase of output voltage (degrees)"
      mask help:
      | This discrete block generates pulses for carrier-based PWM (Pulse Width Modulation), self-commutated IGBTs,GTOs or FETs bridges.
      |
      | Depending on the number of bridge arms selected in the "Generator Mode" parameter, the block can be used either for single-phase or three-phase PWM control.
      mask init:
      | powericon('psbcallbacks',gcb,'Discrete PWM Generator');
      | if Freq==0
      |     Phase=90;
      | end
      | switch GeneratorMode
      | case 1,
      |     Internal_Phase=0;
      |    Signal_PortWidth=1;
      |    Select1_Elements=[1 2];
      |    Select1_PortWidth=2;
      |    Select3_Elements=[1 2];
      |    Select3_PortWidth=4;
      | case 2,
      |     Internal_Phase=0;
      |     Signal_PortWidth=1;
      |     Select1_Elements=[1 2];
      |     Select1_PortWidth=2;
      |     Select3_Elements=[1 2 3 4];
      |     Select3_PortWidth=4;
      | case 3,
      |     Internal_Phase=[0 -2*pi/3 2*pi/3];
      |     Signal_PortWidth=3;
      |     Select1_Elements=[1 4 2 5 3 6];
      |     Select1_PortWidth=6;
      |    Select3_Elements=[1 2 3 4 5 6];
      |    Select3_PortWidth=12;
      | case 4,
      |     Internal_Phase=[0 -2*pi/3 2*pi/3];
      |     Signal_PortWidth=3;
      |     Select1_Elements=[1 4 2 5 3 6];
      |     Select1_PortWidth=6;
      |    Select3_Elements=[1 2 3 4 5 6 7 8 9 10 11 12];
      |    Select3_PortWidth=12;
      | end
      | power_initmask();
      mask Help:
      | The output pulses are a vector (with values=0 or 1). Depending on the selected "Generator Mode", the output vector contains:
      | For a 1-arm  bridge: Two pulses. Pulse 1 is for the upper switch and pulse 2 is for the lower switch.
      | For a 2-arm  bridge: Four pulses. Pulses 1 and 3 are respectively for the upper switches of the first and second arm. Pulses 2 and 4 are for the lower switches.
      | For a 3-arm  bridge: Six pulses. Pulses 1,3 and 5 are respectively for the upper switches of the first,second and third arm. Pulses 2,4 and 6 are for the lower switches.
      | For double 3-arm bridges: Twelve pulses.The first six pulses (pulses 1 to 6) must be sent to the first 3-arm bridge and the last six (pulses 7 to 12) to the second 3-arm bridge.
      | 
      | By selecting "Internal generation" you can can control the modulation index m, frequency and phase of the output voltage  from the internal parameters (m, Freq and Phase). Otherwise, external signals are used for pulse generation. The width of the input vector must be 1 for single phase bridges ( 1-arm or 2-arm)  and 3 for 3-phase bridges  (single or double bridge).
      mask TypeOptions GeneratorMode: 1-arm  bridge (2 pulses) | 2-arm  bridge (4 pulses) | 3-arm  bridge (6 pulses) | Double 3-arm  bridges (12 pulses)
      mask Callback Internal: powericon('psbcallbacks',gcb,'Discrete PWM Generator',[]);
  MI Controller : Subsystem
  Unit Delay4 : UnitDelay  SampleTime=Ts_Power  HasFrameUpgradeWarning=on
  VL-L_1 : Scope  NumInputPorts=2
  Vph_abc : Scope
  Vph_rms_1 : Scope
  u / m : Scope
  Pulses : Outport  VectorParamsAs1DForOutWhenUnconnected=off
  wires:
  MI Controller/2(u / m) -> u / m/1
  Unit Delay4/1 -> Pulses/1
  Discrete PWM Generator1/1(Pulses) -> Unit Delay4/1
  Bus Selector/1 -> Vph_abc/1, MI Controller/1(Vabc)  "<signal1>"
  Bus Selector/2 -> VL-L_1/1  "<signal2>"
  Bus Selector/3 -> VL-L_1/2  "<signal3>"
  Bus Selector/4 -> Vph_rms_1/1  "<signal4>"
  Means/1 -> Bus Selector/1
  MI Controller/1(Vabc_inv) -> Discrete PWM Generator1/1(Uref)

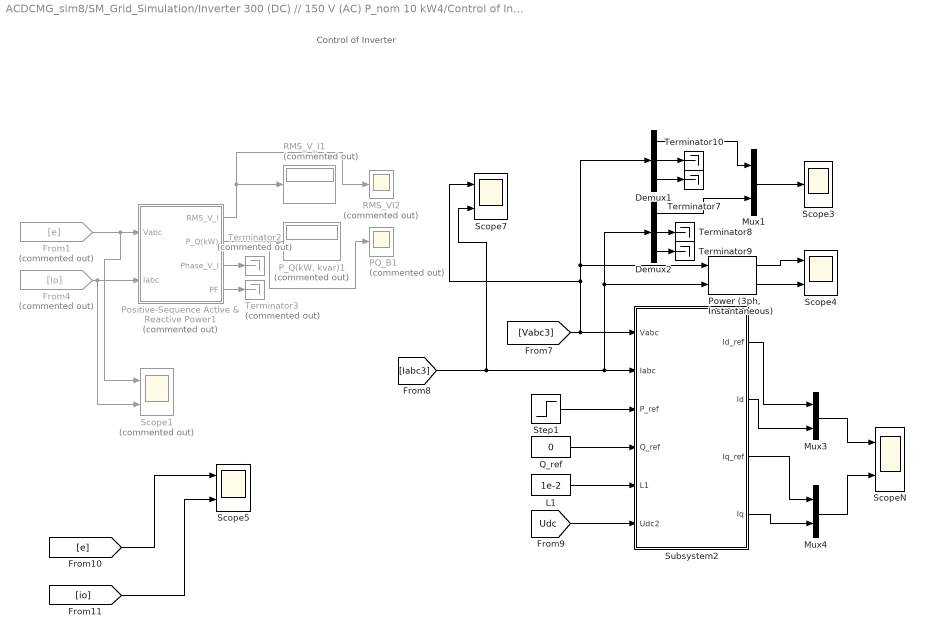
== system ACDCMG_sim8/SM_Grid_Simulation/Inverter 300 (DC) // 150 V (AC) P_nom 10 kW4/Control of Inverter ==
  note: Control of Inverter
  Demux1 : Demux  Outputs=3
  Demux2 : Demux  Outputs=3
  From1 : From  Commented=on  GotoTag=e
      settings: CloseFcn=tagdialog Close
  From4 : From  Commented=on  GotoTag=io
      settings: CloseFcn=tagdialog Close
  L1 : Constant  Value=1e-2
  Mux1 : Mux  Inputs=2
  Mux3 : Mux  Inputs=2
  Mux4 : Mux  Inputs=2
  PQ_B1 : Scope  Commented=on
  "P_Q(kW, kvar)1" : Display  Commented=on
      settings: Format=bank  Decimation=2000
  Positive-Sequence Active & Reactive Power1 : Subsystem  Commented=on  AncestorBlock=|  DialogController=POWERSYS.PowerSysDialog  mask(Discrete 3-phase Positive-Sequence Active & Reactive Power){Freq=60, Par_Vinit=[0 0], Par_Iinit=[0 0], Ts=5e-6}
      | powerlib_extras/Discrete
      | Measurements/Discrete 3-phase 
      | Positive-Sequence 
      | Active & Reactive Power
      mask prompts: Freq "Fundamental frequency (Hz):"; Par_Vinit "Voltage initial input: [ Mag  Phase(degrees) ]"; Par_Iinit "Current initial input: [ Mag  Phase(degrees) ]"; Ts "Sample time:"
      mask help:
      | Measure the three-phase active power P and reactive power Q associated with a periodic set of three-phase voltages and currents which may contain harmonics. P and Q are calculated by evaluating the fundamental values (positive-sequence) of the input voltages and currents with a running window over one cycle of the fundamental frequency.
      |
      | Current flowing into an RL circuit will produce  positive active and reactive powers.
      |
      | Vabc input: Three-phase instantaneous voltage (V)
      | Iabc input: Three-phase instantaneous current (A)
      |
      | Output 1: Vector [Mag_V(V) Mag_I(A)] of the fundamental values of the voltage & current (peak values of the positive-sequence)
      | Output 2: 3-phase PQ measurement vector [P(W) Q (var)] evaluated at the fundamental frequency.
      |
      | For the first cycle of simulation, the outputs are held constant using the values specified by the parameters "Initial input".
      mask init:
      | power_initmask();
      mask Help: This block is part of a subset of blocks in the Extras library that does not have documentation associated with it, other than the block mask description.
      mask Display: disp('')
  "Power (3ph, Instantaneous)" : powerlib_meascontrol/Measurements/Power (3ph, Instantaneous)
  Q_ref : Constant  Value=0
  RMS_VI2 : Scope  Commented=on
  RMS_V_I1 : Display  Commented=on
      settings: Format=bank  Decimation=2000
  Scope1 : Scope  Commented=on  NumInputPorts=2
  Scope3 : Scope
  Scope4 : Scope  NumInputPorts=2
  Scope5 : Scope  NumInputPorts=2
  Scope7 : Scope  NumInputPorts=2
  ScopeN : Scope  NumInputPorts=2
  Step1 : Step  Time=0.07  After=15e3  SampleTime=0
  Subsystem2 : Subsystem  mask{Kp=100, Ki=101, Kd=0}
      mask prompts: Kp "Proportional gain (Kp):"; Ki "Integral gain (Ki):"; Kd "Derivative gain (Kd):"
  Terminator{7..10} (4 alike) : Terminator
  Terminator2 : Terminator  Commented=on
  Terminator3 : Terminator  Commented=on
  wires:
  From4/1 -> Scope1/2, Positive-Sequence Active & Reactive Power1/2(Iabc)
  Positive-Sequence Active & Reactive Power1/2(P_Q(kW)) -> PQ_B1/1, "P_Q(kW, kvar)1"/1
  Positive-Sequence Active & Reactive Power1/4(PF) -> Terminator3/1
  Positive-Sequence Active & Reactive Power1/3(Phase_V_I) -> Terminator2/1
  Positive-Sequence Active & Reactive Power1/1(RMS_V_I) -> RMS_V_I1/1, RMS_VI2/1
  From1/1 -> Scope1/1, Positive-Sequence Active & Reactive Power1/1(Vabc)
  Q_ref/1 -> Subsystem2/4(Q_ref)
  [Vabc3] -> Subsystem2/1(Vabc), Scope7/1, Demux1/1, "Power (3ph, Instantaneous)"/1
  Demux2/3 -> Terminator9/1
  Demux1/2 -> Terminator10/1
  [Udc] -> Subsystem2/6(Udc2)
  Step1/1 -> Subsystem2/3(P_ref)
  Demux2/2 -> Terminator8/1
  "Power (3ph, Instantaneous)"/2 -> Scope4/2
  "Power (3ph, Instantaneous)"/1 -> Scope4/1
  Subsystem2/3(Iq_ref) -> Mux4/1
  Subsystem2/2(Id) -> Mux3/2
  Demux2/1 -> Mux1/2
  Mux1/1 -> Scope3/1
  L1/1 -> Subsystem2/5(L1)
  Mux3/1 -> ScopeN/1
  Subsystem2/4(Iq) -> Mux4/2
  [Iabc3] -> Scope7/2, Demux2/1, "Power (3ph, Instantaneous)"/2, Subsystem2/2(Iabc)
  Subsystem2/1(Id_ref) -> Mux3/1
  Mux4/1 -> ScopeN/2
  Demux1/3 -> Terminator7/1
  Demux1/1 -> Mux1/1
  [io] -> Scope5/2
  [e] -> Scope5/1

== system ACDCMG_sim8/SM_Grid_Simulation/Boost -buck Bi-directional converter 1/Primary Control/PID Orig Boost ==
  error : Inport
  Delay : Delay  DelayLength=1  InitialCondition=0  SampleTime=Ts
  Integrator : Integrator  InitialCondition=0.1  LimitOutput=on  UpperSaturationLimit=0.9  LowerSaturationLimit=0.1
  Ki : Gain  Gain=0.001
  Kp : Gain  Gain=0.000005
  Kp1 : Gain  Gain=60
  Sum1 : Sum  Inputs=|++
  Out1 : Outport  VectorParamsAs1DForOutWhenUnconnected=off
  wires:
  Integrator/1 -> Sum1/2
  Sum1/1 -> Out1/1
  Ki/1 -> Integrator/1
  Kp/1 -> Sum1/1
  error/1 -> Delay/1
  Delay/1 -> Kp1/1
  Kp1/1 -> Kp/1, Ki/1

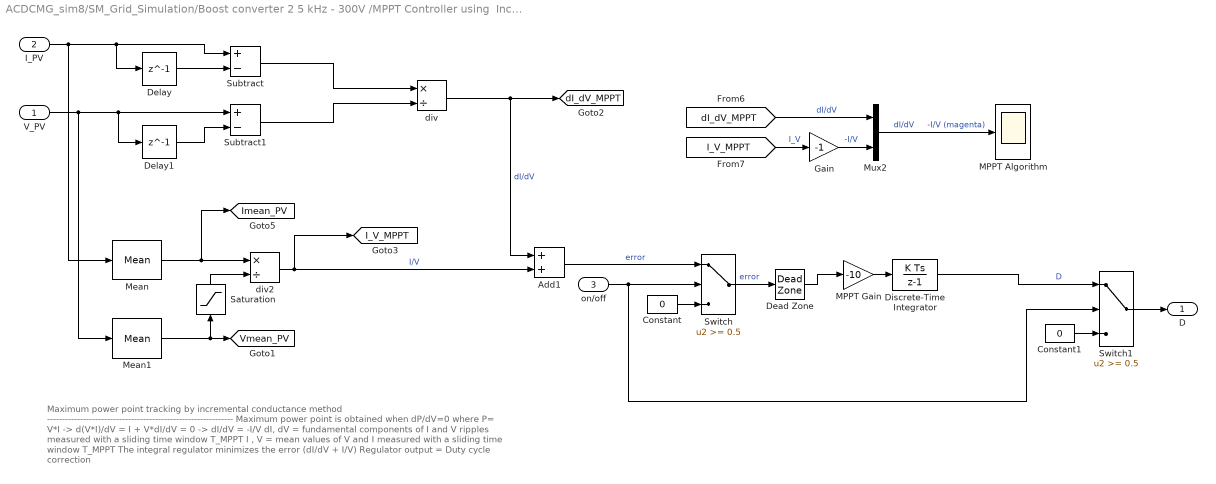
== system ACDCMG_sim8/SM_Grid_Simulation/Boost converter 2 5 kHz - 300V /MPPT Controller using  Incremental Conductance and Integral Regulator  technique /MPPT ==
  note: Maximum power point tracking by incremental conductance method
      | --------------------------------------------------------------
      | Maximum power point is obtained when dP/dV=0  where P= V*I
      | -> d(V*I)/dV = I + V*dI/dV = 0
      | -> dI/dV = -I/V
      |
      | dI, dV  = fundamental components of I and V ripples measured with a sliding time window T_MPPT
      | I , V   = mean values of V and I measured with a sliding time window T_MPPT
      |
      | The integral regulator minimizes the error (dI/dV + I/V)
      | Regulator output = Duty cycle correction
  V_PV : Inport
  I_PV : Inport  Port=2
  on/off : Inport  Port=3
  Add1 : Sum
  Constant : Constant  Value=0
  Constant1 : Constant  Value=0
  Dead Zone : DeadZone  LowerValue=-0.0001  UpperValue=0.0001  SaturateOnIntegerOverflow=on
  Delay : Delay  DelayLength=1  InitialCondition=0  SampleTime=Ts_Power
  Delay1 : Delay  DelayLength=1  InitialCondition=0  SampleTime=Ts_Power
  Discrete-Time Integrator : DiscreteIntegrator  InitialCondition=0.3  SampleTime=Ts_Control  LimitOutput=on  UpperSaturationLimit=0.9  LowerSaturationLimit=0.1  ICPrevOutput=DiscIntNeverNeededParam  ICPrevScaledInput=DiscIntNeverNeededParam
  Gain : Gain  Gain=-1
  MPPT Gain : Gain  Gain=-10
  MPPT Algorithm : Scope
  Mean : powerlib_meascontrol/Measurements/Mean  Freq=5000  Vinit=0  Ts=Ts_Power
  Mean1 : powerlib_meascontrol/Measurements/Mean  Freq=5000  Vinit=0  Ts=Ts_Power
  Mux2 : Mux  Inputs=2
  Saturation : Saturate  UpperLimit=inf  LowerLimit=Vmin_mppt
  Subtract : Sum  Inputs=+-
  Subtract1 : Sum  Inputs=+-
  Switch : Switch  Threshold=0.5
  Switch1 : Switch  Threshold=0.5
  div : Product  Inputs=*/  RndMeth=Zero
  div2 : Product  Inputs=*/  RndMeth=Zero
  D : Outport  VectorParamsAs1DForOutWhenUnconnected=off
  tag scope: I_V_MPPT=global, Imean_PV=global, Vmean_PV=global, dI_dV_MPPT=global
  wires:
  Dead Zone/1 -> MPPT Gain/1
  Switch/1 -> Dead Zone/1  "error"
  Saturation/1 -> div2/2
  Switch1/1 -> D/1
  on/off/1 -> Switch/2, Switch1/2
  Constant1/1 -> Switch1/3
  Constant/1 -> Switch/3
  MPPT Gain/1 -> Discrete-Time Integrator/1
  Add1/1 -> Switch/1  "error"
  div2/1 -> Add1/2, [I_V_MPPT]  "I/V"
  Mean1/1 -> Saturation/1, [Vmean_PV]
  Mean/1 -> div2/1, [Imean_PV]
  div/1 -> [dI_dV_MPPT], Add1/1  "dI/dV"
  V_PV/1 -> Subtract1/1, Delay1/1, Mean1/1
  I_PV/1 -> Subtract/1, Delay/1, Mean/1
  [dI_dV_MPPT] -> Mux2/1  "dI/dV"
  Gain/1 -> Mux2/2  "-I/V"
  Mux2/1 -> MPPT Algorithm/1  "dI/dV     -I/V (magenta)"
  [I_V_MPPT] -> Gain/1  "I_V"
  Delay/1 -> Subtract/2
  Delay1/1 -> Subtract1/2
  Subtract/1 -> div/1
  Subtract1/1 -> div/2
  Discrete-Time Integrator/1 -> Switch1/1  "D"

== system ACDCMG_sim8/SM_Grid_Simulation/Bus_AC//DC3/Battery system/Ripple Calculations ==
  Signal : Inport
  Reset : Inport  Port=2
  0 : Constant  Value=2
  1 : Constant  Value=2
  Display10 : Display
  Display2 : Display
  Mean1 : powerlib_meascontrol/Measurements/Mean  Freq=10  Vinit=0  Ts=0
  MinMax Running Resettable : simulink/Math Operations/MinMax Running Resettable  Function=max  vinit=0.0
  MinMax Running Resettable1 : simulink/Math Operations/MinMax Running Resettable  Function=min  vinit=0.0
  Product : Product
  Product1 : Product
  Sum : Sum  Inputs=|+-
  Sum1 : Sum  Inputs=|-+
  Switch1 : Switch  Criteria=u2 > Threshold
  Switch2 : Switch  Criteria=u2 > Threshold
  Switch3 : Switch  Criteria=u2 > Threshold
  Ripple in Buck : Outport  VectorParamsAs1DForOutWhenUnconnected=off
  Ripple in Boost : Outport  Port=2  VectorParamsAs1DForOutWhenUnconnected=off
  wires:
  1/1 -> Product1/2
  [I_ref] -> Switch2/2, Switch3/2
  Product1/1 -> Switch3/3
  0/1 -> Product/2
  Switch2/1 -> Ripple in Buck/1
  Switch3/1 -> Ripple in Boost/1
  Product/1 -> Switch2/1
  Signal/1 -> Mean1/1, MinMax Running Resettable1/1, MinMax Running Resettable/1
  Switch1/1 -> Sum1/2, Sum/2
  MinMax Running Resettable/1 -> Sum/1, Display2/1
  MinMax Running Resettable1/1 -> Sum1/1, Display10/1
  Sum/1 -> Product/1
  Reset/1 -> Switch1/2, MinMax Running Resettable1/2, MinMax Running Resettable/2
  Sum1/1 -> Product1/1
  Mean1/1 -> Switch1/3

== system ACDCMG_sim8/SM_Grid_Simulation/Bus_AC//DC3/PV system/Pmean ==
  Product : Product  RndMeth=Zero
  Scope : Scope  NumInputPorts=2
  W-kW : Gain  Gain=1/1000
  P : Outport  VectorParamsAs1DForOutWhenUnconnected=off
  V : Outport  Port=2  VectorParamsAs1DForOutWhenUnconnected=off
  wires:
  [Vdc_PV] -> Scope/1, Product/1, V/1
  Product/1 -> W-kW/1
  [Idc_PV] -> Scope/2, Product/2
  W-kW/1 -> P/1  "Pmean_PV (kW)"

== system ACDCMG_sim8/SM_Grid_Simulation/Grid Bi-directional Converter 1.1 300 (DC) // 150 V (AC) P_nom 3kW2/Control of Inverter/Discrete PWM Generator1 ==
  note: Pierre Giroux, Gilbert Sybille
      | Power System Laboratory, IREQ
      | Hydro-Quebec
  note: PWM Generator
  Uref : Inport
  BL4 : Logic  Operator=NOT  Inputs=1
  BL5 : Logic  Operator=NOT  Inputs=1
  Constant : Constant  Value=Internal_Phase
  Constant1 : Constant  Value=Internal
  Data Type Conversion : DataTypeConversion  OutDataTypeStr=double  SaturateOnIntegerOverflow=on  RndMeth=Zero
  Data Type Conversion1 : DataTypeConversion  OutDataTypeStr=boolean  SaturateOnIntegerOverflow=on  RndMeth=Zero
  Data Type Conversion2 : DataTypeConversion  OutDataTypeStr=boolean  SaturateOnIntegerOverflow=on  RndMeth=Zero
  Gain : Gain  Gain=2*pi*Freq  SaturateOnIntegerOverflow=on  OutDataTypeStr=Inherit: Same as input  ParamDataTypeStr=Inherit: Same as input
  Gain2 : Gain  Gain=pi/180  SaturateOnIntegerOverflow=on  OutDataTypeStr=Inherit: Same as input  ParamDataTypeStr=Inherit: Same as input
  Gain3 : Gain  Gain=-1  SaturateOnIntegerOverflow=on  OutDataTypeStr=Inherit: Same as input  ParamDataTypeStr=Inherit: Same as input
  Mux : Mux  Inputs=2
  Mux1 : Mux  Inputs=2
  Mux2 : Mux  Inputs=2
  Product : Product  SaturateOnIntegerOverflow=on  InputSameDT=on  OutDataTypeStr=Inherit: Same as first input
  Relational Operator : RelationalOperator  RndMeth=Nearest  InputSameDT=on
  Relational Operator1 : RelationalOperator  RndMeth=Nearest  InputSameDT=on
  Select1A : Selector  InputPortWidth=Select1_PortWidth  IndexOptions=Index vector (dialog)  Indices=Select1_Elements  OutputSizes=1
  Select1B : Selector  InputPortWidth=Select1_PortWidth  IndexOptions=Index vector (dialog)  Indices=Select1_Elements  OutputSizes=1
  Select3 : Selector  InputPortWidth=Select3_PortWidth  IndexOptions=Index vector (dialog)  Indices=Select3_Elements  OutputSizes=1
  Sum : Sum  Inputs=+++  SaturateOnIntegerOverflow=on  InputSameDT=on  OutDataTypeStr=Inherit: Same as first input
  Switch : Switch  Criteria=u2 > Threshold
  Triangle : simulink/Sources/Repeating Sequence  rep_seq_t=[0 1/Fc/4 3/Fc/4 1/Fc]  rep_seq_y=[0 -1 1 0]
  Trigonometric Function : Trigonometry
  m3 : Constant  Value=Phase
  m4 : Constant  Value=mIndex
  t : DigitalClock  SampleTime=Ts
  Pulses : Outport  VectorParamsAs1DForOutWhenUnconnected=off
  wires:
  Mux2/1 -> Select3/1
  Select1B/1 -> Mux2/2
  Select1A/1 -> Mux2/1
  Mux1/1 -> Select1B/1
  Mux/1 -> Select1A/1
  BL5/1 -> Mux1/2
  BL4/1 -> Mux/2
  Gain3/1 -> Relational Operator1/1
  Triangle/1 -> Relational Operator1/2, Relational Operator/2
  Product/1 -> Switch/1
  Constant1/1 -> Switch/2
  Trigonometric Function/1 -> Product/2
  Sum/1 -> Trigonometric Function/1
  m4/1 -> Product/1
  Constant/1 -> Sum/3
  m3/1 -> Gain2/1
  Gain2/1 -> Sum/2
  Gain/1 -> Sum/1
  t/1 -> Gain/1
  Select3/1 -> Data Type Conversion/1
  Data Type Conversion/1 -> Pulses/1
  Relational Operator/1 -> Data Type Conversion1/1
  Data Type Conversion1/1 -> BL4/1, Mux/1
  Relational Operator1/1 -> Data Type Conversion2/1
  Data Type Conversion2/1 -> BL5/1, Mux1/1
  Switch/1 -> Relational Operator/1, Gain3/1
  Uref/1 -> Switch/3

== system ACDCMG_sim8/SM_Grid_Simulation/Grid Bi-directional Converter 1.1 300 (DC) // 150 V (AC) P_nom 3kW2/Control of Inverter/MI Controller ==
  Vabc : Inport
  Demux : Demux  Commented=on  Outputs=3
  Demux1 : Demux  Outputs=3
  Mux : Mux  Inputs=3
  Mux1 : Mux  Inputs=3
  Mux2 : Mux  Inputs=3
  OP max / min : Subsystem
  Product : Product  RndMeth=Zero
  Product1 : Product  RndMeth=Zero
  Product2 : Product  RndMeth=Zero
  Subsystem : Subsystem
  Subsystem1 : Subsystem
  Terminator : Terminator
  Terminator1 : Terminator  Commented=on
  Terminator2 : Terminator  Commented=on
  Terminator3 : Terminator
  Terminator4 : Terminator  Commented=on
  Vab1 : powerlib_extras/Discrete Measurements/Discrete  RMS value  Commented=on  Freq=60  Mag_Init=0  Ts=20e-6
      settings: SourceProductBaseCode=PS
  Vab5 : powerlib_extras/Discrete Measurements/Discrete  RMS value  Commented=on  Freq=60  Mag_Init=0  Ts=20e-6
      settings: SourceProductBaseCode=PS
  Vab6 : powerlib_extras/Discrete Measurements/Discrete  RMS value  Commented=on  Freq=60  Mag_Init=0  Ts=20e-6
      settings: SourceProductBaseCode=PS
  Vabc_inv : Outport  VectorParamsAs1DForOutWhenUnconnected=off
  u / m : Outport  Port=2  VectorParamsAs1DForOutWhenUnconnected=off
  wires:
  Product/1 -> Mux2/1
  Product1/1 -> Mux2/2
  Product2/1 -> Mux2/3
  Mux1/1 -> u / m/1
  Vabc/1 -> Demux/1
  Demux/1 -> Vab6/1
  Demux/2 -> Vab5/1
  Demux/3 -> Vab1/1
  Demux1/1 -> Product/1, Mux1/1
  Demux1/2 -> Product1/1, Mux1/2
  Demux1/3 -> Product2/1, Mux1/3
  Subsystem/1(Va) -> Product/2
  Subsystem/2(Vb) -> Product1/2
  Subsystem/3(Vc) -> Product2/2
  Mux2/1 -> Vabc_inv/1
  Vab6/1 -> Terminator2/1
  Subsystem1/3(wt) -> Terminator/1
  Subsystem1/1(Frec) -> Terminator3/1
  Subsystem1/2(sin_cos) -> Subsystem/1(sin_cos)
  Mux/1 -> Demux1/1
  OP max / min/1(ctrl) -> Mux/3, Mux/1, Mux/2
  Vab5/1 -> Terminator1/1
  Vab1/1 -> Terminator4/1

== system ACDCMG_sim8/SM_Grid_Simulation/Inverter 300 (DC) // 150 V (AC) P_nom 10 kW4/Control of Inverter/Positive-Sequence Active & Reactive Power1 ==
  note: Discrete 3-phase Positive-Sequence Active & Reactive Power
  note: Pierre Giroux, Gilbert Sybille
      | Power System Simulation Laboratory
      | IREQ, Hydro-Quebc
  Vabc : Inport  PortDimensions=3
  Iabc : Inport  Port=2  PortDimensions=3
  Deg->Rad : Gain  Gain=pi/180  SaturateOnIntegerOverflow=on  OutDataTypeStr=Inherit: Same as input  ParamDataTypeStr=Inherit: Same as input
  Discrete 3-phase Positive-Sequence Fundamental Value (I) : powerlib_extras/Discrete Measurements/Discrete 3-phase Positive-Sequence Fundamental Value  Freq=Freq  Par_Init=Par_Iinit  Ts=Ts
      settings: SourceProductBaseCode=PS
  Discrete 3-phase Positive-Sequence Fundamental Value (V) : powerlib_extras/Discrete Measurements/Discrete 3-phase Positive-Sequence Fundamental Value  Freq=Freq  Par_Init=Par_Vinit  Ts=Ts
      settings: SourceProductBaseCode=PS
  Gain1 : Gain  Gain=3/2  SaturateOnIntegerOverflow=on  OutDataTypeStr=Inherit: Same as input  ParamDataTypeStr=Inherit: Same as input
  Mag->RMS : Gain  Gain=1/sqrt(2)
  Mux1 : Mux  Inputs=2
  Mux2 : Mux  Inputs=2
  Mux3 : Mux  Inputs=2
  Product : Product  SaturateOnIntegerOverflow=on  InputSameDT=on  OutDataTypeStr=Inherit: Same as first input
  Product1 : Product  SaturateOnIntegerOverflow=on  InputSameDT=on  OutDataTypeStr=Inherit: Same as first input
  Product2 : Product  SaturateOnIntegerOverflow=on  InputSameDT=on  OutDataTypeStr=Inherit: Same as first input
  Sum : Sum  Inputs=+-  SaturateOnIntegerOverflow=on  InputSameDT=on  OutDataTypeStr=Inherit: Same as first input
  Trigonometric Function : Trigonometry
  Trigonometric Function1 : Trigonometry  Operator=cos
  W->kW Var->kvar : Gain  Gain=1/1000
  RMS_V_I : Outport
  P_Q(kW) : Outport  Port=2
  Phase_V_I : Outport  Port=3
  PF : Outport  Port=4
  wires:
  Vabc/1 -> Discrete 3-phase Positive-Sequence Fundamental Value (V)/1
  Iabc/1 -> Discrete 3-phase Positive-Sequence Fundamental Value (I)/1
  Discrete 3-phase Positive-Sequence Fundamental Value (V)/2 -> Sum/1, Mux1/1
  Discrete 3-phase Positive-Sequence Fundamental Value (I)/2 -> Sum/2, Mux1/2
  Sum/1 -> Deg->Rad/1
  Deg->Rad/1 -> Trigonometric Function1/1, Trigonometric Function/1
  Trigonometric Function1/1 -> PF/1, Product/2
  Trigonometric Function/1 -> Product1/1
  Mux2/1 -> Gain1/1
  Product/1 -> Mux2/1
  Product1/1 -> Mux2/2
  Product2/1 -> Product/1, Product1/2
  Discrete 3-phase Positive-Sequence Fundamental Value (V)/1 -> Mux3/1, Product2/1
  Discrete 3-phase Positive-Sequence Fundamental Value (I)/1 -> Mux3/2, Product2/2
  Mux1/1 -> Phase_V_I/1
  Mux3/1 -> Mag->RMS/1
  Mag->RMS/1 -> RMS_V_I/1
  Gain1/1 -> W->kW Var->kvar/1
  W->kW Var->kvar/1 -> P_Q(kW)/1
